simulink model "digital_flc"  (R2014a)
settings: Solver=VariableStepDiscrete  StartTime=0.0  StopTime=10.0  RelTol=1e-3
undefined symbols (not defined in the file or in its folder): DiscIntNeverNeededParam
libraries: fuzblock x1
settings Model: Creator=krish  LastModifiedBy=krish

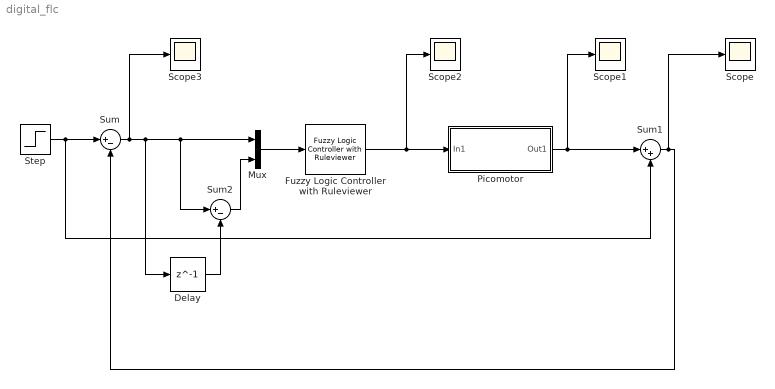
== system digital_flc ==
  Delay : Delay  DelayLength=1  InitialCondition=0
  Fuzzy Logic Controller with Ruleviewer : fuzblock/Fuzzy Logic  Controller  with Ruleviewer  fismatrix='flc_pid2.fis'  Ts=2
  Mux : Mux  Inputs=2
  "Picomotor " : Subsystem
  Scope{,1..3} (4 alike) : Scope
      Scope settings: TimeRange=0.001966153848734442  YMin=0.4783320787422278  YMax=0.4895433515597992  SaveName=ScopeData2
      Scope1 settings: TimeRange=0.001966153848734442  YMin=0.4783320787422278  YMax=0.4895433515597992
      Scope2 settings: TimeRange=0.001966153848734442  YMin=0.4783320787422278  YMax=0.4895433515597992  SaveName=ScopeData3
      Scope3 settings: TimeRange=0.001966153848734442  YMin=0.4783320787422278  YMax=0.4895433515597992  SaveName=ScopeData4
  Step : Step  SampleTime=0
  Sum : Sum  Inputs=|+-
  Sum1 : Sum  Inputs=|++
  Sum2 : Sum  Inputs=|+-
  wires:
  Step/1 -> Sum1/2, Sum/1
  Sum/1 -> Scope3/1, Delay/1, Sum2/1, Mux/1
  Mux/1 -> Fuzzy Logic Controller with Ruleviewer/1
  Sum1/1 -> Scope/1, Sum/2
  Fuzzy Logic Controller with Ruleviewer/1 -> Scope2/1, "Picomotor "/1(In1)
  "Picomotor "/1(Out1) -> Scope1/1, Sum1/1
  Delay/1 -> Sum2/2
  Sum2/1 -> Mux/2

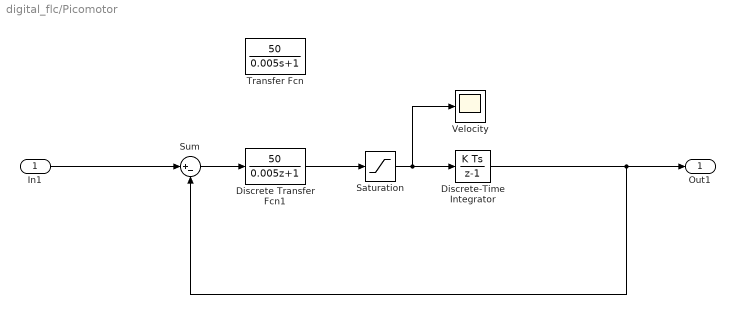
== system digital_flc/Picomotor  ==
  In1 : Inport  OutMin=-6  OutMax=6
  Discrete Transfer Fcn1 : DiscreteTransferFcn  Numerator=[50]  Denominator=[0.005 1]
  Discrete-Time Integrator : DiscreteIntegrator  ICPrevOutput=DiscIntNeverNeededParam  ICPrevScaledInput=DiscIntNeverNeededParam
  Saturation : Saturate
  Sum : Sum  Inputs=|+-
  Transfer Fcn : TransferFcn  Numerator=[50]  Denominator=[0.005 1]
  Velocity : Scope
      settings: TimeRange=10
  Out1 : Outport
  wires:
  In1/1 -> Sum/1
  Saturation/1 -> Discrete-Time Integrator/1, Velocity/1
  Sum/1 -> Discrete Transfer Fcn1/1
  Discrete Transfer Fcn1/1 -> Saturation/1
  Discrete-Time Integrator/1 -> Sum/2, Out1/1
